simulink model "gm_HDLRx_vs"  (R2024a)
settings: Solver=FixedStepDiscrete  StartTime=0.0  StopTime=stopTime  RelTol=1e-3
undefined symbols (not defined in the file or in its folder): channelBitsPerSubcarrier, channelCyclicPrefixLen, channelOFDMSamples, channelScramblerInit, clk, clk_enable, decimatorDelay, decimatorFilter, fPHY, fs, headerBitsPerFec, headerBitsPerSubcarrier, headerCyclicPrefixLen, headerOFDMSamples, headerScramblerInit, lowerbound, N, numDataCarriers, payloadBitsPerFec, payloadScramblerInit, preambleBitsPerSubcarrier, preambleCyclicPrefixLen, preambleFirstPartOFDMSamples, preambleScramblerInit, preambleSecondPartOFDMSamples, QAM, reset_x, upperbound
libraries: hdlsllib x133, hdlmdlgenlib x132, simulink x8, whdlutilities x8, whdlmod x4, dspsrcs4 x2, whdledac x2, commhdlcrc x1, dsphdlfiltering2 x1, dsphdlsigops2 x1, vivadosimlib x1, HDL_ieee_8021513 x1
(part 1 of 4)
settings Model: Creator=cotti  LastModifiedBy=cotti
settings OptimizationCC: BlockReduction=off  ConditionallyExecuteInputs=off  DefaultParameterBehavior=Inlined  InheritOutputTypeSmallerThanSingle=on
settings DebuggingCC: AlgebraicLoopMsg=error  ArtificialAlgebraicLoopMsg=error  InheritedTsInSrcMsg=none  SingleTaskRateTransMsg=error  UnconnectedInputMsg=warning  UnconnectedOutputMsg=warning  UnconnectedLineMsg=warning
settings HardwareCC: ProdBitPerPointer=32  ProdBitPerSizeT=32  ProdBitPerPtrDiffT=32  ProdLargestAtomicFloat=None  ProdIntDivRoundTo=Undefined  ProdEndianess=Unspecified  ProdWordSize=32  ProdHWDeviceType=ASIC/FPGA->ASIC/FPGA  TargetBitPerLong=64  TargetBitPerPointer=64  TargetBitPerSizeT=64  TargetBitPerPtrDiffT=64  TargetLongLongMode=on  TargetIntDivRoundTo=Zero  TargetEndianess=LittleEndian  TargetWordSize=64  TargetHWDeviceType=Custom Processor->MATLAB Host Computer  ProdEqTarget=off

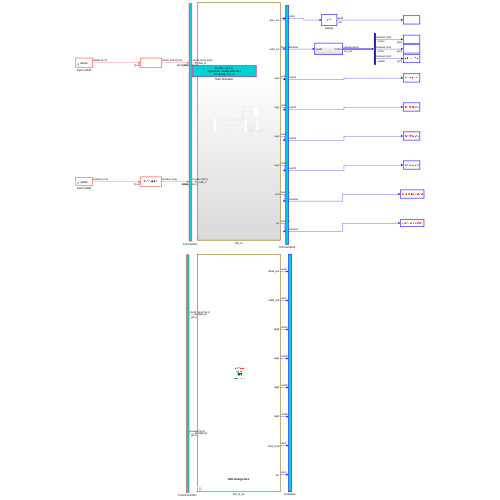
[thumbnail: Simulink's stored preview of the top-level diagram]
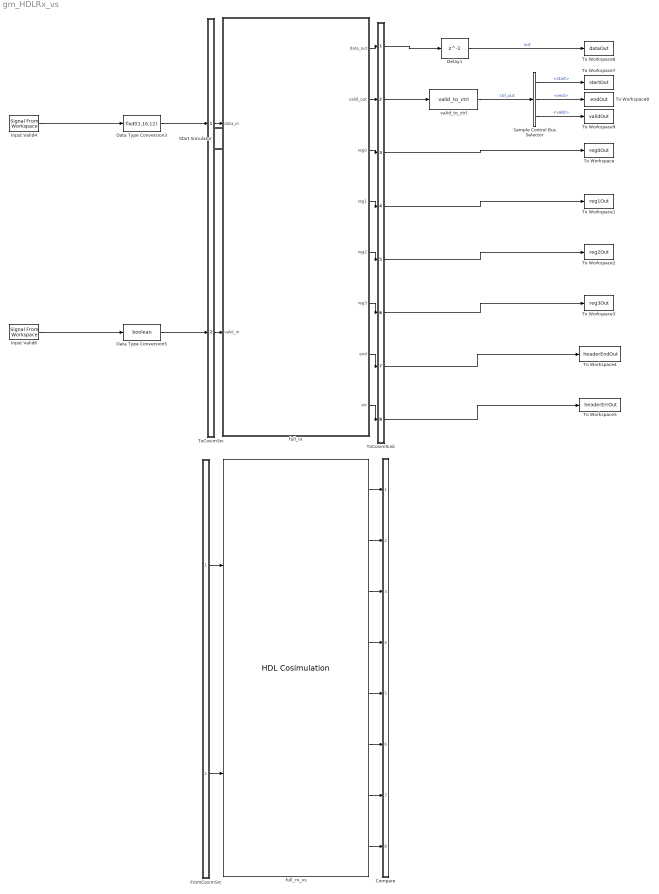
== system gm_HDLRx_vs ==
  Compare : Subsystem
      mask Display: disp('')
  Data Type Conversion3 : DataTypeConversion  OutDataTypeStr=fixdt(1,16,12)  SaturateOnIntegerOverflow=off  RndMeth=Floor
  Data Type Conversion5 : DataTypeConversion  OutDataTypeStr=boolean  SaturateOnIntegerOverflow=off  RndMeth=Floor
  Delay1 : Delay  DelayLength=1  InitialCondition=0  UseCircularBuffer=on
  FromCosimSrc : Subsystem
      mask Display: disp('')
  Input Valid4 : dspsrcs4/Signal From Workspace  X=dataIn  Ts=1/fs  nsamps=1  OutputAfterFinalValue=Setting to zero  ignoreOrWarnInputAndFrameLengths=off  OutputFrames=off
  Input Valid6 : dspsrcs4/Signal From Workspace  X=validIn  Ts=1/fs  nsamps=1  OutputAfterFinalValue=Setting to zero  ignoreOrWarnInputAndFrameLengths=off  OutputFrames=off
  Sample Control Bus Selector : whdlutilities/Sample Control Bus Selector  OutputSignals=start,end,valid
  Start Simulator : Subsystem
      settings: OpenFcn=|
      | cosimDirName = pwd;
      | cd 'hdl_prj/hdlsrc/HDLRx';
      | [s,r] = system('vivado -mode batch -source gm_HDLRx_vs.tcl','-echo');
      | cd (cosimDirName);
      | clear cosimDirName;
      | if s
      |    error('Failed to create Vivado HDL design DLL using script gm_HDLRx_vs.tcl.');
      | end
      mask Display: disp('Double-click to\nregenerate Vivado HDL DLL\nfor design full_rx')
  To Workspace : ToWorkspace  VariableName=reg0Out  SampleTime=4/fPHY
      settings: Save2DSignal=2-D array (concatenate along first dimension)
  To Workspace1 : ToWorkspace  VariableName=reg1Out  SampleTime=4/fPHY
      settings: Save2DSignal=2-D array (concatenate along first dimension)
  To Workspace2 : ToWorkspace  VariableName=reg2Out  SampleTime=4/fPHY
      settings: Save2DSignal=2-D array (concatenate along first dimension)
  To Workspace3 : ToWorkspace  VariableName=reg3Out  SampleTime=4/fPHY
      settings: Save2DSignal=2-D array (concatenate along first dimension)
  To Workspace4 : ToWorkspace  VariableName=headerEndOut  SampleTime=4/fPHY
      settings: Save2DSignal=2-D array (concatenate along first dimension)
  To Workspace5 : ToWorkspace  VariableName=headerErrOut  SampleTime=4/fPHY
      settings: Save2DSignal=2-D array (concatenate along first dimension)
  To Workspace6 : ToWorkspace  VariableName=dataOut  SampleTime=4/fPHY
      settings: Save2DSignal=2-D array (concatenate along first dimension)
  To Workspace7 : ToWorkspace  VariableName=startOut  SampleTime=4/fPHY
      settings: Save2DSignal=2-D array (concatenate along first dimension)
  To Workspace8 : ToWorkspace  VariableName=endOut  SampleTime=4/fPHY
      settings: Save2DSignal=2-D array (concatenate along first dimension)
  To Workspace9 : ToWorkspace  VariableName=validOut  SampleTime=4/fPHY
      settings: Save2DSignal=2-D array (concatenate along first dimension)
  ToCosimSink : Subsystem
      mask Display: disp('')
  ToCosimSrc : Subsystem
      mask Display: disp('')
  full_rx : Subsystem
  full_rx_vs : vivadosimlib/HDL Cosimulation  PortPaths=/full_rx/data_in;/full_rx/valid_in;/full_rx/data_out;/full_rx/valid_out;/full_rx/reg0;/full_rx/reg1;/full_rx/reg2;/full_rx/reg3;/full_rx/end_rsvd;/full_rx/err  PortModes=[1 1 2 2 2 2 2 2 2 2 ]  PortTimes=[-1 -1 8.0000000000000001673804866410277814026130727143026888370513916016e-08 8.0000000000000001673804866410277814026130727143026888370513916016e-08 8.0000000000000001673804866410277814026130727143026888370513916016e-08 8.0000000000000001673804866410277814026130727143026888370513916016e-08 8.0000000000000001673804866410277814026130727143026888370513916016e-08 8.0000000000000001673804866410277814026130727143026888370513916016e-08 8.0000000000000001673804866410277814026130727143026888370513916016e-08 8.0000000000000001673804866410277814026130727143026888370513916016e-08 ]  PortSigns=[-1 -1 0 0 0 0 0 0 0 0 ]  PortFracLengths=[0,0,0,0,0,0,0,0,0,0]  PortWordLengths=[-1,-1,8,1,32,32,32,32,1,1]  PortHDLWordSizes=[16,1,8,1,32,32,32,32,1,1]  CommLocal=on  CommSharedMemory=on  CommPortNumber=4449  CommShowInfo=on  ClockPaths=clk;clk_enable;reset_x;  ClockModes=[2 4 3]  ClockTimes=[1e-08 3.7e-08 2.7e-08]  TclPostSimCommand="puts \"done\""  TimingMode=ns  TimingScaleFactor=1000000000  idxCellArray={'UNUSED_VAR'}  CosimBypass=Full Simulation  AllowDirectFeedthrough=on  ProductName=EDA Simulator Link VS  RunAutoTimescale=off  HdlClocks=0  PreRunTime=40  PreRunTimeUnit=ns
  valid_to_ctrl : HDL_ieee_8021513/valid_to_ctrl  SystemSampleTime=-1  VariantActivationTime=update diagram  AllowFlexibleInterface=on  Latency=0  AutoFrameSizeCalculation=off
      settings: SourceProductName=HDL IEEE 8021513
  wires:
  Sample Control Bus Selector/3 -> To Workspace9/1  "<valid>"
  Sample Control Bus Selector/1 -> To Workspace7/1  "<start>"
  Delay1/1 -> To Workspace6/1  "out"
  valid_to_ctrl/1 -> Sample Control Bus Selector/1  "ctrl_out"
  Sample Control Bus Selector/2 -> To Workspace8/1  "<end>"
  Input Valid6/1 -> Data Type Conversion5/1
  Input Valid4/1 -> Data Type Conversion3/1
  ToCosimSrc/1(out1) -> full_rx/1(data_in)
  ToCosimSrc/2(out2) -> full_rx/2(valid_in)
  full_rx/1(data_out) -> ToCosimSink/1(in1)
  full_rx/2(valid_out) -> ToCosimSink/2(in2)
  full_rx/3(reg0) -> ToCosimSink/3(in3)
  full_rx/4(reg1) -> ToCosimSink/4(in4)
  full_rx/5(reg2) -> ToCosimSink/5(in5)
  full_rx/6(reg3) -> ToCosimSink/6(in6)
  full_rx/7(end) -> ToCosimSink/7(in7)
  full_rx/8(err) -> ToCosimSink/8(in8)
  Data Type Conversion3/1 -> ToCosimSrc/1(in1)
  Data Type Conversion5/1 -> ToCosimSrc/2(in2)
  ToCosimSink/1(out1) -> Delay1/1
  ToCosimSink/2(out2) -> valid_to_ctrl/1
  ToCosimSink/3(out3) -> To Workspace/1
  ToCosimSink/4(out4) -> To Workspace1/1
  ToCosimSink/5(out5) -> To Workspace2/1
  ToCosimSink/6(out6) -> To Workspace3/1
  ToCosimSink/7(out7) -> To Workspace4/1
  ToCosimSink/8(out8) -> To Workspace5/1
  FromCosimSrc/1(out1) -> full_rx_vs/1
  FromCosimSrc/2(out2) -> full_rx_vs/2
  full_rx_vs/1 -> Compare/1(in1)
  full_rx_vs/2 -> Compare/2(in2)
  full_rx_vs/3 -> Compare/3(in3)
  full_rx_vs/4 -> Compare/4(in4)
  full_rx_vs/5 -> Compare/5(in5)
  full_rx_vs/6 -> Compare/6(in6)
  full_rx_vs/7 -> Compare/7(in7)
  full_rx_vs/8 -> Compare/8(in8)

== system gm_HDLRx_vs/Compare ==
  in1 : Inport
  in2 : Inport  Port=2
  in3 : Inport  Port=3
  in4 : Inport  Port=4
  in5 : Inport  Port=5
  in6 : Inport  Port=6
  in7 : Inport  Port=7
  in8 : Inport  Port=8
  Assert_data_out : Subsystem
      settings: LibrarySourceBlock=hdlmdlgenlib/AssertEq
  Assert_end : Subsystem
      settings: LibrarySourceBlock=hdlmdlgenlib/AssertEq
  Assert_err : Subsystem
      settings: LibrarySourceBlock=hdlmdlgenlib/AssertEq
  Assert_reg0 : Subsystem
      settings: LibrarySourceBlock=hdlmdlgenlib/AssertEq
  Assert_reg1 : Subsystem
      settings: LibrarySourceBlock=hdlmdlgenlib/AssertEq
  Assert_reg2 : Subsystem
      settings: LibrarySourceBlock=hdlmdlgenlib/AssertEq
  Assert_reg3 : Subsystem
      settings: LibrarySourceBlock=hdlmdlgenlib/AssertEq
  Assert_valid_out : Subsystem
      settings: LibrarySourceBlock=hdlmdlgenlib/AssertEq
  CleanupScopes : Subsystem
      settings: OpenFcn=|
      | blkName = gcb; %self block
      | idx = regexp(blkName, '/CleanupScopes$', 'once');
      | blkParent = blkName(1:idx-1);
      | blks=find_system(blkParent, 'LookUnderMasks', 'all','blocktype', 'Scope');
      | for itr = 1:length(blks)
      | 	 hScopeCfg = get_param(blks{itr},'ScopeConfiguration');
      | 	 hScopeCfg.Visible = ~ hScopeCfg.Visible;
      | end
      | drawnow;
      mask Display: fprintf(message('hdlcoder:cosim:vnl_dblclick').getString());
  Enable : Subsystem
      settings: OpenFcn=|
      | blkName = gcb;
      | idx = regexp(blkName, '/Enable$', 'once');
      | blkParent = blkName(1:idx-1);
      | blks=find_system(blkParent, 'LookUnderMasks', 'all','blocktype', 'Assertion');
      | e = get_param(blks{1}, 'Enabled');
      | if strcmp(e, 'on'), f= 'off';, else, f = 'on';, end
      | for ii=1:length(blks), set_param(blks{ii}, 'Enabled', f);, end
      | set_param(gcb, 'MaskDisplay',['fprintf(message(''hdlcoder:cosim:vnl_dblclick_assertions'',','''',upper(e),'''',').getString())']);
      mask Display: fprintf(message('hdlcoder:cosim:vnl_dblclick_assertions','OFF').getString());
  wires:
  [out2] -> Assert_valid_out/2(dut)
  in2/1 -> Assert_valid_out/1(cosim)
  in4/1 -> Assert_reg1/1(cosim)
  [out4] -> Assert_reg1/2(dut)
  in5/1 -> Assert_reg2/1(cosim)
  [out5] -> Assert_reg2/2(dut)
  [out1] -> Assert_data_out/2(dut)
  [out7] -> Assert_end/2(dut)
  in6/1 -> Assert_reg3/1(cosim)
  [out3] -> Assert_reg0/2(dut)
  [out6] -> Assert_reg3/2(dut)
  [out8] -> Assert_err/2(dut)
  in8/1 -> Assert_err/1(cosim)
  in7/1 -> Assert_end/1(cosim)
  in1/1 -> Assert_data_out/1(cosim)
  in3/1 -> Assert_reg0/1(cosim)

== system gm_HDLRx_vs/FromCosimSrc ==
  out1 : Outport
  out2 : Outport  Port=2
  wires:
  [in2] -> out2/1
  [in1] -> out1/1

== system gm_HDLRx_vs/Start Simulator ==

== system gm_HDLRx_vs/ToCosimSink ==
  in1 : Inport
  in2 : Inport  Port=2
  in3 : Inport  Port=3
  in4 : Inport  Port=4
  in5 : Inport  Port=5
  in6 : Inport  Port=6
  in7 : Inport  Port=7
  in8 : Inport  Port=8
  out1 : Outport
  out2 : Outport  Port=2
  out3 : Outport  Port=3
  out4 : Outport  Port=4
  out5 : Outport  Port=5
  out6 : Outport  Port=6
  out7 : Outport  Port=7
  out8 : Outport  Port=8
  tag scope: out1=global, out2=global, out3=global, out4=global, out5=global, out6=global, out7=global, out8=global
  wires:
  in1/1 -> out1/1, [out1]
  in2/1 -> out2/1, [out2]
  in3/1 -> out3/1, [out3]
  in4/1 -> out4/1, [out4]
  in5/1 -> out5/1, [out5]
  in6/1 -> out6/1, [out6]
  in7/1 -> out7/1, [out7]
  in8/1 -> out8/1, [out8]

== system gm_HDLRx_vs/ToCosimSrc ==
  in1 : Inport
  in2 : Inport  Port=2
  out1 : Outport
  out2 : Outport  Port=2
  tag scope: in1=global, in2=global
  wires:
  in1/1 -> out1/1, [in1]
  in2/1 -> out2/1, [in2]

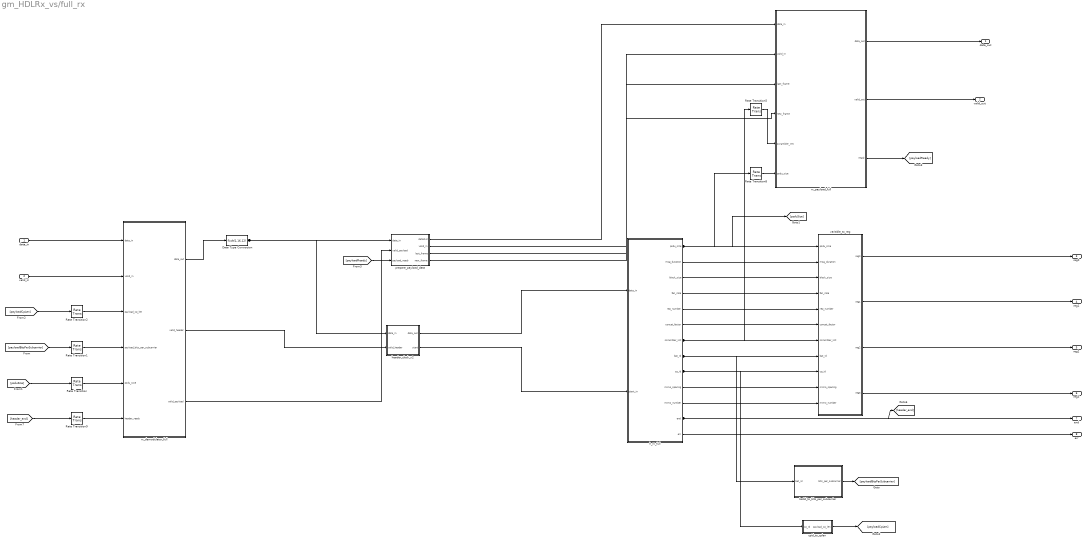
== system gm_HDLRx_vs/full_rx ==
  data_in : Inport  OutDataTypeStr=fixdt(1, 16, 12)  SampleTime=1e-08
  valid_in : Inport  Port=2  OutDataTypeStr=boolean  SampleTime=1e-08
  Data Type Conversion : DataTypeConversion  OutDataTypeStr=fixdt(1,16,12)  SaturateOnIntegerOverflow=off  RndMeth=Floor
  Rate Transition{,1..2,9} (4 alike) : RateTransition  OutPortSampleTime=1/fPHY
  Rate Transition5 : RateTransition  OutPortSampleTime=1/(2*fPHY)
  Rate Transition8 : RateTransition  OutPortSampleTime=1/(2*fPHY)
  batid_to_bits_per_subcarrier : Subsystem
  cpid_to_cplen : Subsystem
  h_rx_full : Subsystem
  header_clock_x2 : Subsystem
  prepare_payload_data : Subsystem
  rx_demodulator_full : Subsystem
  rx_payload_full : Subsystem
  variable_to_reg : Subsystem
  data_out : Outport  SampleTime=8e-08
  valid_out : Outport  Port=2  SampleTime=8e-08
  reg0 : Outport  Port=3  SampleTime=8e-08
  reg1 : Outport  Port=4  SampleTime=8e-08
  reg2 : Outport  Port=5  SampleTime=8e-08
  reg3 : Outport  Port=6  SampleTime=8e-08
  end : Outport  Port=7  SampleTime=8e-08
  err : Outport  Port=8  SampleTime=8e-08
  wires:
  variable_to_reg/4(reg3) -> reg3/1
  variable_to_reg/3(reg2) -> reg2/1
  variable_to_reg/2(reg1) -> reg1/1
  variable_to_reg/1(reg0) -> reg0/1
  rx_payload_full/3(ready) -> [payloadReady]
  rx_payload_full/2(valid_out) -> valid_out/1
  rx_payload_full/1(data_out) -> data_out/1
  rx_demodulator_full/3(valid_payload) -> prepare_payload_data/2(valid_payload)
  rx_demodulator_full/2(valid_header) -> header_clock_x2/2(valid_header)
  rx_demodulator_full/1(data_out) -> Data Type Conversion/1
  prepare_payload_data/4(new_frame) -> rx_payload_full/4(new_frame)
  prepare_payload_data/3(last_frame) -> rx_payload_full/3(last_frame)
  prepare_payload_data/2(valid_in) -> rx_payload_full/2(valid_in)
  prepare_payload_data/1(dataOut) -> rx_payload_full/1(data_in)
  header_clock_x2/2(start) -> h_rx_full/2(start_in)
  header_clock_x2/1(data_out) -> h_rx_full/1(data_in)
  h_rx_full/13(err) -> err/1
  h_rx_full/12(end) -> end/1, [header_end]
  h_rx_full/11(mimo_number) -> variable_to_reg/11(mimo_number)
  h_rx_full/10(mimo_spacing) -> variable_to_reg/10(mimo_spacing)
  h_rx_full/9(cp_id) -> cpid_to_cplen/1(cp_id), variable_to_reg/9(cp_id)
  h_rx_full/8(bat_id) -> batid_to_bits_per_subcarrier/1(bat_id), variable_to_reg/8(bat_id)
  h_rx_full/7(scrambler_init) -> variable_to_reg/7(scrambler_init), Rate Transition5/1
  h_rx_full/6(concat_factor) -> variable_to_reg/6(concat_factor)
  h_rx_full/5(rep_number) -> variable_to_reg/5(rep_number)
  h_rx_full/4(fec_rate) -> variable_to_reg/4(fec_rate)
  h_rx_full/3(block_size) -> variable_to_reg/3(block_size)
  h_rx_full/2(msg_duration) -> variable_to_reg/2(msg_duration)
  h_rx_full/1(psdu_size) -> variable_to_reg/1(psdu_size), [psduSize], Rate Transition8/1
  cpid_to_cplen/1(payload_cp_len) -> [payloadCpLen]
  batid_to_bits_per_subcarrier/1(bits_per_subcarrier) -> [payloadBitsPerSubcarrier]
  Rate Transition9/1 -> rx_demodulator_full/6(header_ready)
  Rate Transition8/1 -> rx_payload_full/6(psdu_size)
  Rate Transition5/1 -> rx_payload_full/5(scrambler_init)
  Rate Transition2/1 -> rx_demodulator_full/3(payload_cp_len)
  Rate Transition1/1 -> rx_demodulator_full/4(payload_bits_per_subcarrier)
  Rate Transition/1 -> rx_demodulator_full/5(psdu_size)
  [header_end] -> Rate Transition9/1
  [payloadReady] -> prepare_payload_data/3(payload_ready)
  [payloadCpLen] -> Rate Transition2/1
  [psduSize] -> Rate Transition/1
  [payloadBitsPerSubcarrier] -> Rate Transition1/1
  Data Type Conversion/1 -> prepare_payload_data/1(data_in), header_clock_x2/1(data_in)
  valid_in/1 -> rx_demodulator_full/2(valid_in)
  data_in/1 -> rx_demodulator_full/1(data_in)

== system gm_HDLRx_vs/Compare/Assert_data_out ==
  cosim : Inport
  dut : Inport  Port=2
  AssertEq : Assertion
  Compare To Zero : simulink/Logic and Bit Operations/Compare To Zero  relop===  OutDataTypeStr=boolean
  Relational Operator : RelationalOperator  Operator===  OutDataTypeStr=boolean  InputSameDT=off
  compare: data_out : Scope  NumInputPorts=3
  wires:
  Compare To Zero/1 -> compare: data_out/3  "err"
  Relational Operator/1 -> Compare To Zero/1, AssertEq/1
  cosim/1 -> compare: data_out/1, Relational Operator/1  "cosim"
  dut/1 -> compare: data_out/2, Relational Operator/2  "dut ref"

== system gm_HDLRx_vs/Compare/Assert_end ==
  cosim : Inport
  dut : Inport  Port=2
  AssertEq : Assertion
  Compare To Zero : simulink/Logic and Bit Operations/Compare To Zero  relop===  OutDataTypeStr=boolean
  Relational Operator : RelationalOperator  Operator===  OutDataTypeStr=boolean  InputSameDT=off
  compare: end : Scope  NumInputPorts=3
  wires:
  Compare To Zero/1 -> compare: end/3  "err"
  Relational Operator/1 -> Compare To Zero/1, AssertEq/1
  cosim/1 -> compare: end/1, Relational Operator/1  "cosim"
  dut/1 -> compare: end/2, Relational Operator/2  "dut ref"

== system gm_HDLRx_vs/Compare/Assert_err ==
  cosim : Inport
  dut : Inport  Port=2
  AssertEq : Assertion
  Compare To Zero : simulink/Logic and Bit Operations/Compare To Zero  relop===  OutDataTypeStr=boolean
  Relational Operator : RelationalOperator  Operator===  OutDataTypeStr=boolean  InputSameDT=off
  compare: err : Scope  NumInputPorts=3
  wires:
  Compare To Zero/1 -> compare: err/3  "err"
  Relational Operator/1 -> Compare To Zero/1, AssertEq/1
  cosim/1 -> compare: err/1, Relational Operator/1  "cosim"
  dut/1 -> compare: err/2, Relational Operator/2  "dut ref"

== system gm_HDLRx_vs/Compare/Assert_reg0 ==
  cosim : Inport
  dut : Inport  Port=2
  AssertEq : Assertion
  Compare To Zero : simulink/Logic and Bit Operations/Compare To Zero  relop===  OutDataTypeStr=boolean
  Relational Operator : RelationalOperator  Operator===  OutDataTypeStr=boolean  InputSameDT=off
  compare: reg0 : Scope  NumInputPorts=3
  wires:
  Compare To Zero/1 -> compare: reg0/3  "err"
  Relational Operator/1 -> Compare To Zero/1, AssertEq/1
  cosim/1 -> compare: reg0/1, Relational Operator/1  "cosim"
  dut/1 -> compare: reg0/2, Relational Operator/2  "dut ref"

== system gm_HDLRx_vs/Compare/Assert_reg1 ==
  cosim : Inport
  dut : Inport  Port=2
  AssertEq : Assertion
  Compare To Zero : simulink/Logic and Bit Operations/Compare To Zero  relop===  OutDataTypeStr=boolean
  Relational Operator : RelationalOperator  Operator===  OutDataTypeStr=boolean  InputSameDT=off
  compare: reg1 : Scope  NumInputPorts=3
  wires:
  Compare To Zero/1 -> compare: reg1/3  "err"
  Relational Operator/1 -> Compare To Zero/1, AssertEq/1
  cosim/1 -> compare: reg1/1, Relational Operator/1  "cosim"
  dut/1 -> compare: reg1/2, Relational Operator/2  "dut ref"

== system gm_HDLRx_vs/Compare/Assert_reg2 ==
  cosim : Inport
  dut : Inport  Port=2
  AssertEq : Assertion
  Compare To Zero : simulink/Logic and Bit Operations/Compare To Zero  relop===  OutDataTypeStr=boolean
  Relational Operator : RelationalOperator  Operator===  OutDataTypeStr=boolean  InputSameDT=off
  compare: reg2 : Scope  NumInputPorts=3
  wires:
  Compare To Zero/1 -> compare: reg2/3  "err"
  Relational Operator/1 -> Compare To Zero/1, AssertEq/1
  cosim/1 -> compare: reg2/1, Relational Operator/1  "cosim"
  dut/1 -> compare: reg2/2, Relational Operator/2  "dut ref"

== system gm_HDLRx_vs/Compare/Assert_reg3 ==
  cosim : Inport
  dut : Inport  Port=2
  AssertEq : Assertion
  Compare To Zero : simulink/Logic and Bit Operations/Compare To Zero  relop===  OutDataTypeStr=boolean
  Relational Operator : RelationalOperator  Operator===  OutDataTypeStr=boolean  InputSameDT=off
  compare: reg3 : Scope  NumInputPorts=3
  wires:
  Compare To Zero/1 -> compare: reg3/3  "err"
  Relational Operator/1 -> Compare To Zero/1, AssertEq/1
  cosim/1 -> compare: reg3/1, Relational Operator/1  "cosim"
  dut/1 -> compare: reg3/2, Relational Operator/2  "dut ref"

== system gm_HDLRx_vs/Compare/Assert_valid_out ==
  cosim : Inport
  dut : Inport  Port=2
  AssertEq : Assertion
  Compare To Zero : simulink/Logic and Bit Operations/Compare To Zero  relop===  OutDataTypeStr=boolean
  Relational Operator : RelationalOperator  Operator===  OutDataTypeStr=boolean  InputSameDT=off
  compare: valid_out : Scope  NumInputPorts=3
  wires:
  Compare To Zero/1 -> compare: valid_out/3  "err"
  Relational Operator/1 -> Compare To Zero/1, AssertEq/1
  cosim/1 -> compare: valid_out/1, Relational Operator/1  "cosim"
  dut/1 -> compare: valid_out/2, Relational Operator/2  "dut ref"

== system gm_HDLRx_vs/Compare/CleanupScopes ==

== system gm_HDLRx_vs/Compare/Enable ==

== system gm_HDLRx_vs/full_rx/batid_to_bits_per_subcarrier ==
  note: Remember that "bat_id" is LSB first.
  note: De momento, el valor de BATID va a coincidir con el valor de la cantidad de bits por subcarrier.
  bat_id : Inport  OutDataTypeStr=fixdt(0, 1, 0)  PortDimensions=[5]  SampleTime=8e-08
  Bit Concat : hdlsllib/Logic and Bit Operations/Bit Concat  numInputs=4
  From{,1..3} (4 alike) : hdlmdlgenlib/Buffer
  Goto{1..4} (4 alike) : hdlmdlgenlib/Buffer
  bat_id_4_term4 : Terminator
  t : Demux  Outputs=5
  bits_per_subcarrier : Outport  SampleTime=8e-08
  wires:
  t/5 -> bat_id_4_term4/1
  t/4 -> Goto1/1
  t/3 -> Goto2/1
  t/2 -> Goto3/1
  t/1 -> Goto4/1
  Goto1/1 -> From3/1
  Goto2/1 -> From2/1
  Goto3/1 -> From1/1
  Goto4/1 -> From/1
  From3/1 -> Bit Concat/1
  From2/1 -> Bit Concat/2
  From1/1 -> Bit Concat/3
  From/1 -> Bit Concat/4
  Bit Concat/1 -> bits_per_subcarrier/1
  bat_id/1 -> t/1

== system gm_HDLRx_vs/full_rx/cpid_to_cplen ==
  cp_id : Inport  OutDataTypeStr=fixdt(0, 1, 0)  PortDimensions=[3]  SampleTime=8e-08
  Bits to Word : hdlsllib/Logic and Bit Operations/Bits to Word
  Constant3 : Constant  Value=N/32  OutDataTypeStr=fixdt(0,4,0)  SampleTime=-1
  Data Type Conversion : DataTypeConversion  OutDataTypeStr=fixdt(0,1,0)  SaturateOnIntegerOverflow=off  RndMeth=Floor
  Delay1 : Delay  DelayLength=1  InitialCondition=0  UseCircularBuffer=on
  Product : Product  OutDataTypeStr=uint8
  payload_cp_len : Outport  SampleTime=8e-08
  wires:
  Product/1 -> Delay1/1
  Delay1/1 -> payload_cp_len/1
  Data Type Conversion/1 -> Bits to Word/1
  Constant3/1 -> Product/1
  Bits to Word/1 -> Product/2
  cp_id/1 -> Data Type Conversion/1

== system gm_HDLRx_vs/full_rx/h_rx_full ==
  data_in : Inport  OutDataTypeStr=fixdt(1, 16, 12)  SampleTime=1e-08
  start_in : Inport  Port=2  OutDataTypeStr=boolean  SampleTime=1e-08
  Data Type Conversion : DataTypeConversion  OutDataTypeStr=int8  SaturateOnIntegerOverflow=off  RndMeth=Floor
  Data Type Conversion1 : DataTypeConversion  OutDataTypeStr=boolean  SaturateOnIntegerOverflow=off  RndMeth=Floor
  LDPC_Deco_Hc_12H : whdledac/LDPC Decoder  ParityCheckMatrix=Hc_12H  BlockSize=14  Algorithm=Min-sum  ScalingFactor=0.75  Termination=Max  SpecifyInputs=Property  NumIterations=ldpcDecoderMaxNumberIterations  MaxNumIterations=8  ParityCheckStatus=off  SimulateUsing=Code generation
  LDPC_Deco_Hc_12H_term2 : Terminator
  Rate Transition : RateTransition  OutPortSampleTimeOpt=Multiple of input port sample time  OutPortSampleTimeMultiple=8
  h_crc_rx : Subsystem
  h_remove_repetition : Subsystem
  h_scrambler : Subsystem
  h_separate : Subsystem
  psdu_size : Outport  SampleTime=8e-08
  msg_duration : Outport  Port=2  SampleTime=8e-08
  block_size : Outport  Port=3  SampleTime=8e-08
  fec_rate : Outport  Port=4  SampleTime=8e-08
  rep_number : Outport  Port=5  SampleTime=8e-08
  concat_factor : Outport  Port=6  SampleTime=8e-08
  scrambler_init : Outport  Port=7  SampleTime=8e-08
  bat_id : Outport  Port=8  SampleTime=8e-08
  cp_id : Outport  Port=9  SampleTime=8e-08
  mimo_spacing : Outport  Port=10  SampleTime=8e-08
  mimo_number : Outport  Port=11  SampleTime=8e-08
  end : Outport  Port=12  SampleTime=8e-08
  err : Outport  Port=13  SampleTime=8e-08
  wires:
  h_separate/12(end) -> end/1
  h_separate/11(mimo_number) -> mimo_number/1
  h_separate/10(mimo_spacing) -> mimo_spacing/1
  h_separate/9(cp_id) -> cp_id/1
  h_separate/8(bat_id) -> bat_id/1
  h_separate/7(scrambler_init) -> scrambler_init/1
  h_separate/6(concat_factor) -> concat_factor/1
  h_separate/5(rep_number) -> rep_number/1
  h_separate/4(fec_rate) -> fec_rate/1
  h_separate/3(block_size) -> block_size/1
  h_separate/2(msg_duration) -> msg_duration/1
  h_separate/1(psdu_size) -> psdu_size/1
  h_scrambler/2(ctrl_out) -> h_crc_rx/2(ctrl_in)
  h_scrambler/1(data_out) -> h_crc_rx/1(data_in)
  h_remove_repetition/2(ctrl_out) -> LDPC_Deco_Hc_12H/2
  h_remove_repetition/1(data_out) -> LDPC_Deco_Hc_12H/1
  h_crc_rx/3(err) -> Rate Transition/1
  h_crc_rx/2(ctrl_out) -> h_separate/2(ctrl_in)
  h_crc_rx/1(data_out) -> h_separate/1(data_in)
  Rate Transition/1 -> err/1
  LDPC_Deco_Hc_12H/3 -> LDPC_Deco_Hc_12H_term2/1
  LDPC_Deco_Hc_12H/2 -> h_scrambler/2(ctrl_in)
  LDPC_Deco_Hc_12H/1 -> h_scrambler/1(data_in)
  Data Type Conversion1/1 -> h_remove_repetition/2(start_in)
  Data Type Conversion/1 -> h_remove_repetition/1(data_in)
  start_in/1 -> Data Type Conversion1/1
  data_in/1 -> Data Type Conversion/1

== system gm_HDLRx_vs/full_rx/header_clock_x2 ==
  data_in : Inport  OutDataTypeStr=fixdt(1, 16, 12)  PortDimensions=[4 1]  SampleTime=2e-08
  valid_header : Inport  Port=2  OutDataTypeStr=boolean  PortDimensions=1  SampleTime=2e-08
  Serializer1D : hdlsllib/HDL Operations/Serializer1D  Ratio=2  IdleCycles=0  validIn=on  startOut=off  validOut=on  inputDataDimensions=2  inputSampleTime=2e-08  inputSignalType=real
  concatenate : Concatenate  Mode=Multidimensional array  ConcatenateDimension=2
  data_in_0_term0 : Terminator
  data_in_1_term1 : Terminator
  rising_edge_detector : Subsystem
  t : Demux
  data_out : Outport  SampleTime=1e-08
  start : Outport  Port=2  SampleTime=1e-08
  wires:
  t/4 -> concatenate/2
  t/3 -> concatenate/1
  t/2 -> data_in_1_term1/1
  t/1 -> data_in_0_term0/1
  rising_edge_detector/1(Out) -> start/1
  concatenate/1 -> Serializer1D/1
  Serializer1D/2 -> rising_edge_detector/1(In)
  Serializer1D/1 -> data_out/1
  valid_header/1 -> Serializer1D/2
  data_in/1 -> t/1

== system gm_HDLRx_vs/full_rx/prepare_payload_data ==
  note: Note_ this delay makes sure that the fifo always has data, and is not emptied in the middle of an LDPC block
  data_in : Inport  OutDataTypeStr=fixdt(1, 16, 12)  PortDimensions=[4 1]  SampleTime=2e-08
  valid_payload : Inport  Port=2  OutDataTypeStr=boolean  PortDimensions=1  SampleTime=2e-08
  payload_ready : Inport  Port=3  OutDataTypeStr=boolean  PortDimensions=1  SampleTime=1e-08
  Delay : Delay  DelayLength=1  InitialCondition=0  UseCircularBuffer=on
  Delay2 : Delay  DelayLength=1000  InitialCondition=0  UseCircularBuffer=on
  HDL FIFO : hdlsllib/HDL RAMs/HDL FIFO  fifo_size=65536  mode=Classic  ratio=1  push_msg=Error  pop_msg=Error  show_empty=on  show_full=off  show_num=off  LabelModeActiveChoice_Mode=Classic  rst_port=off
  Logical Operator2 : Logic  IconShape=distinctive  AllPortsSameDT=off  OutDataTypeStr=boolean
  Logical Operator3 : Logic  Operator=NOT  IconShape=distinctive  AllPortsSameDT=off  OutDataTypeStr=boolean
  Rate Transition3 : RateTransition  OutPortSampleTime=1/(2*fPHY)
  Rate Transition4 : RateTransition  OutPortSampleTime=1/(2*fPHY)
  falling_edge_detector : Subsystem
  payload_clock_x2 : Subsystem
  rising_edge_detector : Subsystem
  dataOut : Outport  SampleTime=1e-08
  valid_in : Outport  Port=2  SampleTime=1e-08
  last_frame : Outport  Port=3  SampleTime=1e-08
  new_frame : Outport  Port=4  SampleTime=1e-08
  wires:
  rising_edge_detector/1(Out) -> Rate Transition3/1
  payload_clock_x2/2(valid_out) -> HDL FIFO/2
  payload_clock_x2/1(data_out) -> HDL FIFO/1
  falling_edge_detector/1(out) -> Delay2/1
  Rate Transition4/1 -> new_frame/1
  Rate Transition3/1 -> last_frame/1
  Logical Operator3/1 -> Logical Operator2/1
  Logical Operator2/1 -> HDL FIFO/3, Delay/1
  HDL FIFO/2 -> rising_edge_detector/1(In), falling_edge_detector/1(in), Logical Operator3/1
  HDL FIFO/1 -> dataOut/1
  Delay2/1 -> Rate Transition4/1
  Delay/1 -> valid_in/1
  payload_ready/1 -> Logical Operator2/2
  valid_payload/1 -> payload_clock_x2/2(valid_in)
  data_in/1 -> payload_clock_x2/1(data_in)

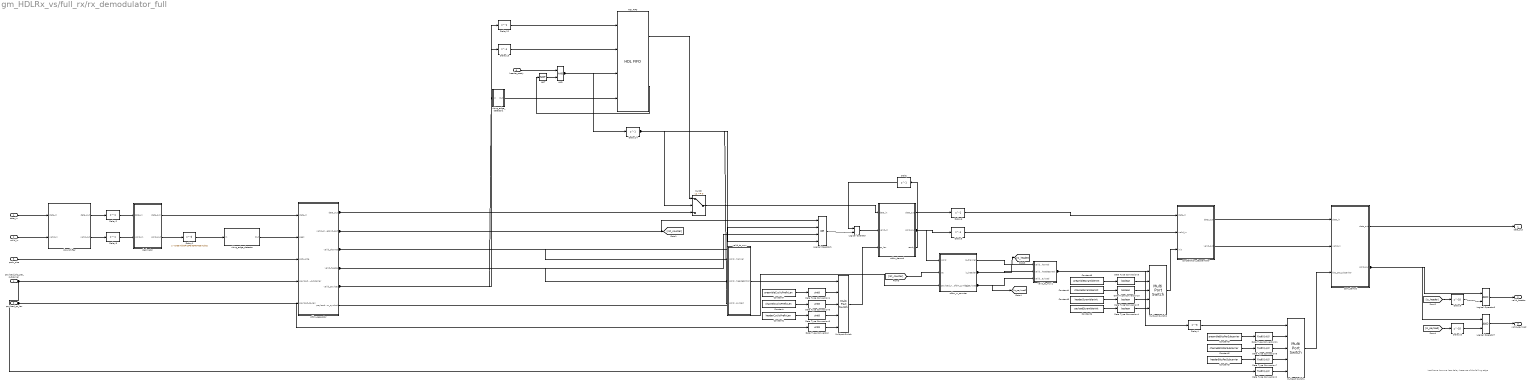
== system gm_HDLRx_vs/full_rx/rx_demodulator_full ==
  note: Last frame has one less delay because of the falling edge
  data_in : Inport  OutDataTypeStr=fixdt(1, 16, 12)  SampleTime=1e-08
  valid_in : Inport  Port=2  OutDataTypeStr=boolean  SampleTime=1e-08
  payload_cp_len : Inport  Port=3  OutDataTypeStr=uint8  SampleTime=2e-08
  payload_bits_per_subcarrier : Inport  Port=4  OutDataTypeStr=fixdt(0, 4, 0)  SampleTime=2e-08
  psdu_size : Inport  Port=5  OutDataTypeStr=fixdt(0, 1, 0)  PortDimensions=[24]  SampleTime=2e-08
  header_ready : Inport  Port=6  OutDataTypeStr=boolean  SampleTime=2e-08
  AND : Logic  IconShape=distinctive  AllPortsSameDT=off  OutDataTypeStr=boolean
  Constant : Constant  Value=channelCyclicPrefixLen  OutDataTypeStr=uint8  SampleTime=-1
  Constant1 : Constant  Value=headerCyclicPrefixLen  OutDataTypeStr=uint8  SampleTime=-1
  Constant2 : Constant  Value=channelBitsPerSubcarrier  OutDataTypeStr=uint8  SampleTime=-1
  Constant3 : Constant  Value=headerBitsPerSubcarrier  OutDataTypeStr=uint8  SampleTime=-1
  Constant4 : Constant  Value=channelScramblerInit  OutDataTypeStr=uint8  SampleTime=-1
  Constant5 : Constant  Value=headerScramblerInit  OutDataTypeStr=uint8  SampleTime=-1
  Constant6 : Constant  Value=payloadScramblerInit  OutDataTypeStr=uint8  SampleTime=-1
  Constant7 : Constant  Value=preambleCyclicPrefixLen  OutDataTypeStr=uint8  SampleTime=-1
  Constant8 : Constant  Value=preambleScramblerInit  OutDataTypeStr=uint8  SampleTime=-1
  Constant9 : Constant  Value=preambleBitsPerSubcarrier  OutDataTypeStr=uint8  SampleTime=-1
  Data Type Conversion{,1,5..6} (4 alike) : DataTypeConversion  OutDataTypeStr=uint8  SaturateOnIntegerOverflow=off  RndMeth=Floor
  Data Type Conversion{3..4,9..10} (4 alike) : DataTypeConversion  OutDataTypeStr=boolean  SaturateOnIntegerOverflow=off  RndMeth=Floor
  Data Type Conversion{2,7..8,11} (4 alike) : DataTypeConversion  OutDataTypeStr=fixdt(0,4,0)  SaturateOnIntegerOverflow=off  RndMeth=Floor
  Delay{,2..3,5..6,12..14} (8 alike) : Delay  DelayLength=1  InitialCondition=0  UseCircularBuffer=on
  Delay1 : Delay  DelayLength=preambleFirstPartOFDMSamples  InitialCondition=0  UseCircularBuffer=on
  Delay10 : Delay  DelayLength=10  InitialCondition=0  UseCircularBuffer=on
  Delay4 : Delay  DelayLength=3  InitialCondition=0  UseCircularBuffer=on
  Delay9 : Delay  DelayLength=10  InitialCondition=0  UseCircularBuffer=on
  HDL FIFO : hdlsllib/HDL RAMs/HDL FIFO  fifo_size=8192  mode=Classic  ratio=1  push_msg=Error  pop_msg=Error  show_empty=on  show_full=off  show_num=off  LabelModeActiveChoice_Mode=Classic  rst_port=on
  Logical Operator : Logic  IconShape=distinctive  AllPortsSameDT=off  OutDataTypeStr=boolean
  Logical Operator1 : Logic  Operator=OR  Inputs=4  IconShape=distinctive  AllPortsSameDT=off  OutDataTypeStr=boolean
  Logical Operator6 : Logic  IconShape=distinctive  AllPortsSameDT=off  OutDataTypeStr=boolean
  Logical Operator7 : Logic  IconShape=distinctive  AllPortsSameDT=off  OutDataTypeStr=boolean
  Multiport Switch : MultiPortSwitch  DataPortOrder=Zero-based contiguous  Inputs=4  zeroidx=on  OutDataTypeStr=uint8  SaturateOnIntegerOverflow=off  InputSameDT=off
  Multiport Switch1 : MultiPortSwitch  DataPortOrder=Zero-based contiguous  Inputs=4  zeroidx=on  OutDataTypeStr=fixdt(0, 4, 0)  SaturateOnIntegerOverflow=off  InputSameDT=off
  Multiport Switch2 : MultiPortSwitch  DataPortOrder=Zero-based contiguous  Inputs=4  zeroidx=on  SaturateOnIntegerOverflow=off  InputSameDT=off
  NOT : Logic  Operator=NOT  IconShape=distinctive  AllPortsSameDT=off  OutDataTypeStr=boolean
  Switch : Switch  Criteria=u2 ~= 0  OutDataTypeStr=fixdt(1, 16, 12)  SaturateOnIntegerOverflow=off  InputSameDT=off
  constellation_descrambler : Subsystem
  decimator : Subsystem
  downshifter : Subsystem
  ofdm_demod : Subsystem
  ofdm_rx_counter : Subsystem
  ofdm_separator : Subsystem
  qam_demod : Subsystem
  rising_edge_detector : Subsystem
  rising_edge_detector1 : Subsystem
  valid_to_mux : Subsystem
  valid_to_mux1 : Subsystem
  data_out : Outport  SampleTime=2e-08
  valid_header : Outport  Port=2  SampleTime=2e-08
  valid_payload : Outport  Port=3  SampleTime=2e-08
  wires:
  valid_to_mux1/1(control) -> Delay4/1, Multiport Switch2/1
  valid_to_mux/1(control) -> Multiport Switch/1
  rising_edge_detector1/1(Out) -> HDL FIFO/4
  rising_edge_detector/1(Out) -> ofdm_separator/2(peak)
  qam_demod/2(valid_out) -> Logical Operator6/1, Logical Operator7/1
  qam_demod/1(data_out) -> data_out/1
  ofdm_separator/6(payload_num_ofdm_symbols) -> ofdm_rx_counter/3(payload_num_ofdm_symbols)
  ofdm_separator/5(valid_payload) -> rising_edge_detector1/1(In), Delay13/1
  ofdm_separator/4(valid_header) -> valid_to_mux/2(valid_header), Logical Operator1/3
  ofdm_separator/3(valid_channel) -> valid_to_mux/1(valid_channel), Logical Operator1/2
  ofdm_separator/2(valid_preamble_second_part) -> [rst_counter], Logical Operator1/1
  ofdm_separator/1(data_out) -> Delay12/1, Switch/3
  ofdm_rx_counter/3(is_payload) -> valid_to_mux1/3(valid_payload), [is_payload]
  ofdm_rx_counter/2(is_header) -> valid_to_mux1/2(valid_header), [is_header]
  ofdm_rx_counter/1(is_channel) -> valid_to_mux1/1(valid_channel)
  ofdm_demod/3(ready) -> Delay/1
  ofdm_demod/2(valid_out) -> ofdm_rx_counter/1(valid), Delay5/1
  ofdm_demod/1(data_out) -> Delay6/1
  downshifter/2(valid_out) -> Delay3/1
  downshifter/1(data_out) -> Delay2/1
  decimator/2(valid_out) -> Delay1/1
  decimator/1(data_out) -> ofdm_separator/1(data_in)
  constellation_descrambler/2(valid_out) -> qam_demod/2(valid_in)
  constellation_descrambler/1(data_out) -> qam_demod/1(data_in)
  Switch/1 -> ofdm_demod/1(data_in)
  NOT/1 -> AND/2
  Multiport Switch2/1 -> constellation_descrambler/3(init)
  Multiport Switch1/1 -> qam_demod/3(bits_per_subcarrier)
  Multiport Switch/1 -> ofdm_demod/3(cp_len)
  Logical Operator7/1 -> valid_payload/1
  Logical Operator6/1 -> valid_header/1
  Logical Operator1/1 -> Logical Operator/2
  Logical Operator/1 -> ofdm_demod/2(valid_in)
  HDL FIFO/2 -> NOT/1
  HDL FIFO/1 -> Switch/1
  [is_payload] -> Delay10/1
  [rst_counter] -> ofdm_rx_counter/2(rst)
  [is_header] -> Delay9/1
  Delay9/1 -> Logical Operator6/2
  Delay6/1 -> constellation_descrambler/1(data_in)
  Delay5/1 -> constellation_descrambler/2(valid_in)
  Delay4/1 -> Multiport Switch1/1
  Delay3/1 -> decimator/2(valid_in)
  Delay2/1 -> decimator/1(data_in)
  Delay14/1 -> valid_to_mux/3(valid_payload), Logical Operator1/4, Switch/2
  Delay13/1 -> HDL FIFO/2
  Delay12/1 -> HDL FIFO/1
  Delay10/1 -> Logical Operator7/2
  Delay1/1 -> rising_edge_detector/1(In)
  Delay/1 -> Logical Operator/1
  Data Type Conversion9/1 -> Multiport Switch2/4
  Data Type Conversion8/1 -> Multiport Switch1/3
  Data Type Conversion7/1 -> Multiport Switch1/4
  Data Type Conversion6/1 -> Multiport Switch/3
  Data Type Conversion5/1 -> Multiport Switch/4
  Data Type Conversion4/1 -> Multiport Switch2/5
  Data Type Conversion3/1 -> Multiport Switch2/2
  Data Type Conversion2/1 -> Multiport Switch1/5
  Data Type Conversion11/1 -> Multiport Switch1/2
  Data Type Conversion10/1 -> Multiport Switch2/3
  Data Type Conversion1/1 -> Multiport Switch/2
  Data Type Conversion/1 -> Multiport Switch/5
  Constant9/1 -> Data Type Conversion11/1
  Constant8/1 -> Data Type Conversion3/1
  Constant7/1 -> Data Type Conversion1/1
  Constant6/1 -> Data Type Conversion4/1
  Constant5/1 -> Data Type Conversion9/1
  Constant4/1 -> Data Type Conversion10/1
  Constant3/1 -> Data Type Conversion7/1
  Constant2/1 -> Data Type Conversion8/1
  Constant1/1 -> Data Type Conversion5/1
  Constant/1 -> Data Type Conversion6/1
  AND/1 -> HDL FIFO/3, Delay14/1
  header_ready/1 -> AND/1
  psdu_size/1 -> ofdm_separator/3(psdu_size)
  payload_bits_per_subcarrier/1 -> ofdm_separator/4(payload_bits_per_subcarrier), Data Type Conversion2/1
  payload_cp_len/1 -> ofdm_separator/5(payload_cp_len), Data Type Conversion/1
  valid_in/1 -> downshifter/2(valid_in)
  data_in/1 -> downshifter/1(data_in)

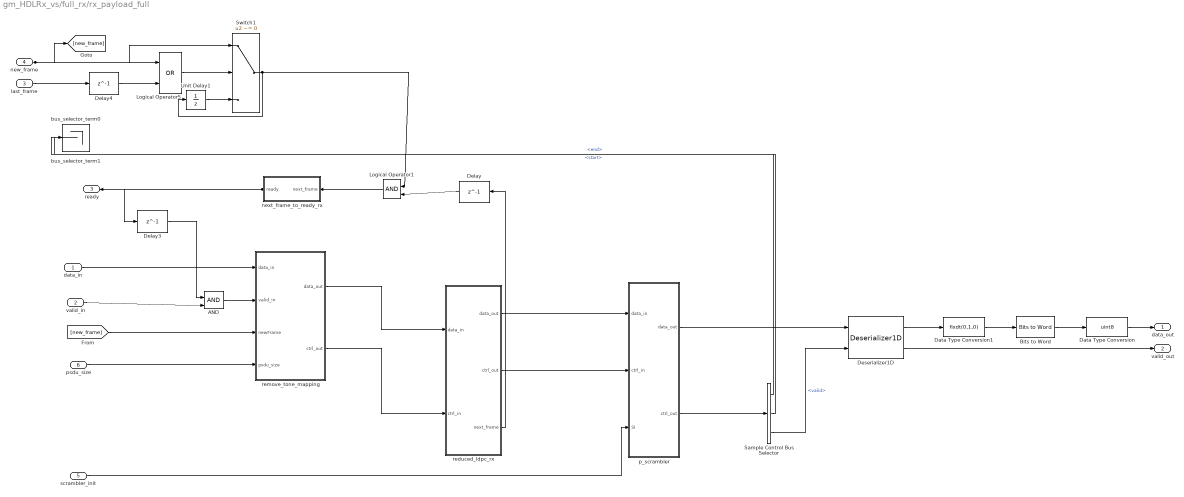
== system gm_HDLRx_vs/full_rx/rx_payload_full ==
  data_in : Inport  OutDataTypeStr=fixdt(1, 16, 12)  SampleTime=1e-08
  valid_in : Inport  Port=2  OutDataTypeStr=boolean  SampleTime=1e-08
  last_frame : Inport  Port=3  OutDataTypeStr=boolean  SampleTime=1e-08
  new_frame : Inport  Port=4  OutDataTypeStr=boolean  SampleTime=1e-08
  scrambler_init : Inport  Port=5  OutDataTypeStr=fixdt(0, 1, 0)  PortDimensions=[4]  SampleTime=1e-08
  psdu_size : Inport  Port=6  OutDataTypeStr=fixdt(0, 1, 0)  PortDimensions=[24]  SampleTime=1e-08
  AND : Logic  IconShape=distinctive  AllPortsSameDT=off  OutDataTypeStr=boolean
  Bits to Word : hdlsllib/Logic and Bit Operations/Bits to Word
  Data Type Conversion : DataTypeConversion  OutDataTypeStr=uint8  SaturateOnIntegerOverflow=off  RndMeth=Floor
  Data Type Conversion1 : DataTypeConversion  OutDataTypeStr=fixdt(0,1,0)  SaturateOnIntegerOverflow=off  RndMeth=Floor
  Delay : Delay  DelayLength=1  InitialCondition=0  UseCircularBuffer=on
  Delay3 : Delay  DelayLength=1  InitialCondition=0  UseCircularBuffer=on
  Delay4 : Delay  DelayLength=1  InitialCondition=0  UseCircularBuffer=on
  Deserializer1D : hdlsllib/HDL Operations/Deserializer1D  Ratio=8  IdleCycles=0  InitialCondition=0  startIn=off  validIn=on  validOut=on  inputDataDimensions=-1  inputSampleTime=-1  inputSignalType=auto
  Logical Operator1 : Logic  IconShape=distinctive  AllPortsSameDT=off  OutDataTypeStr=boolean
  Logical Operator5 : Logic  Operator=OR  IconShape=distinctive  AllPortsSameDT=off  OutDataTypeStr=boolean
  Sample Control Bus Selector : whdlutilities/Sample Control Bus Selector  OutputSignals=start,end,valid
  Switch1 : Switch  Criteria=u2 ~= 0  OutDataTypeStr=boolean  SaturateOnIntegerOverflow=off  InputSameDT=off
  Unit Delay1 : UnitDelay  SampleTime=-1  HasFrameUpgradeWarning=on
  bus_selector_term0 : Terminator
  bus_selector_term1 : Terminator
  next_frame_to_ready_rx : Subsystem
  p_scrambler : Subsystem
  reduced_ldpc_rx : Subsystem
  remove_tone_mapping : Subsystem
  data_out : Outport  SampleTime=8e-08
  valid_out : Outport  Port=2  SampleTime=8e-08
  ready : Outport  Port=3  SampleTime=1e-08
  wires:
  remove_tone_mapping/2(ctrl_out) -> reduced_ldpc_rx/2(ctrl_in)
  remove_tone_mapping/1(data_out) -> reduced_ldpc_rx/1(data_in)
  reduced_ldpc_rx/3(next_frame) -> Delay/1
  reduced_ldpc_rx/2(ctrl_out) -> p_scrambler/2(ctrl_in)
  reduced_ldpc_rx/1(data_out) -> p_scrambler/1(data_in)
  p_scrambler/2(ctrl_out) -> Sample Control Bus Selector/1
  p_scrambler/1(data_out) -> Deserializer1D/1
  next_frame_to_ready_rx/1(ready) -> ready/1, Delay3/1
  Unit Delay1/1 -> Switch1/3
  Switch1/1 -> Unit Delay1/1, Logical Operator1/1
  Sample Control Bus Selector/3 -> Deserializer1D/2  "<valid>"
  Sample Control Bus Selector/2 -> bus_selector_term1/1  "<end>"
  Sample Control Bus Selector/1 -> bus_selector_term0/1  "<start>"
  Logical Operator5/1 -> Switch1/2
  Logical Operator1/1 -> next_frame_to_ready_rx/1(next_frame)
  [new_frame] -> remove_tone_mapping/3(newFrame)
  Deserializer1D/2 -> valid_out/1
  Deserializer1D/1 -> Data Type Conversion1/1
  Delay4/1 -> Logical Operator5/2
  Delay3/1 -> AND/1
  Delay/1 -> Logical Operator1/2
  Data Type Conversion1/1 -> Bits to Word/1
  Data Type Conversion/1 -> data_out/1
  Bits to Word/1 -> Data Type Conversion/1
  AND/1 -> remove_tone_mapping/2(valid_in)
  psdu_size/1 -> remove_tone_mapping/4(psdu_size)
  scrambler_init/1 -> p_scrambler/3(SI)
  new_frame/1 -> [new_frame], Logical Operator5/1, Switch1/1
  last_frame/1 -> Delay4/1
  valid_in/1 -> AND/2
  data_in/1 -> remove_tone_mapping/1(data_in)

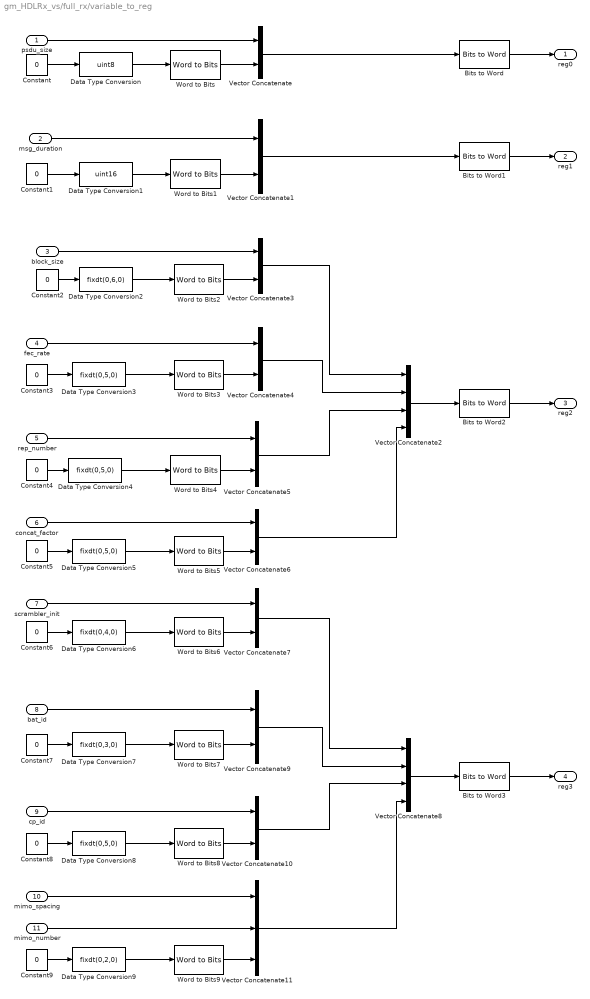
== system gm_HDLRx_vs/full_rx/variable_to_reg ==
  psdu_size : Inport  OutDataTypeStr=fixdt(0, 1, 0)  PortDimensions=[24]  SampleTime=8e-08
  msg_duration : Inport  Port=2  OutDataTypeStr=fixdt(0, 1, 0)  PortDimensions=[16]  SampleTime=8e-08
  block_size : Inport  Port=3  OutDataTypeStr=fixdt(0, 1, 0)  PortDimensions=[2]  SampleTime=8e-08
  fec_rate : Inport  Port=4  OutDataTypeStr=fixdt(0, 1, 0)  PortDimensions=[3]  SampleTime=8e-08
  rep_number : Inport  Port=5  OutDataTypeStr=fixdt(0, 1, 0)  PortDimensions=[3]  SampleTime=8e-08
  concat_factor : Inport  Port=6  OutDataTypeStr=fixdt(0, 1, 0)  PortDimensions=[3]  SampleTime=8e-08
  scrambler_init : Inport  Port=7  OutDataTypeStr=fixdt(0, 1, 0)  PortDimensions=[4]  SampleTime=8e-08
  bat_id : Inport  Port=8  OutDataTypeStr=fixdt(0, 1, 0)  PortDimensions=[5]  SampleTime=8e-08
  cp_id : Inport  Port=9  OutDataTypeStr=fixdt(0, 1, 0)  PortDimensions=[3]  SampleTime=8e-08
  mimo_spacing : Inport  Port=10  OutDataTypeStr=fixdt(0, 1, 0)  PortDimensions=[3]  SampleTime=8e-08
  mimo_number : Inport  Port=11  OutDataTypeStr=fixdt(0, 1, 0)  PortDimensions=[3]  SampleTime=8e-08
  Bits to Word{,1..3} (4 alike) : hdlsllib/Logic and Bit Operations/Bits to Word
  Constant : Constant  Value=0  OutDataTypeStr=uint8  SampleTime=-1
  Constant1 : Constant  Value=0  OutDataTypeStr=uint16  SampleTime=-1
  Constant2 : Constant  Value=0  OutDataTypeStr=fixdt(0,6,0)  SampleTime=-1
  Constant{3..5,8} (4 alike) : Constant  Value=0  OutDataTypeStr=fixdt(0,5,0)  SampleTime=-1
  Constant6 : Constant  Value=0  OutDataTypeStr=fixdt(0,4,0)  SampleTime=-1
  Constant7 : Constant  Value=0  OutDataTypeStr=fixdt(0,3,0)  SampleTime=-1
  Constant9 : Constant  Value=0  OutDataTypeStr=fixdt(0,2,0)  SampleTime=-1
  Data Type Conversion : DataTypeConversion  OutDataTypeStr=uint8  SaturateOnIntegerOverflow=off  RndMeth=Floor
  Data Type Conversion1 : DataTypeConversion  OutDataTypeStr=uint16  SaturateOnIntegerOverflow=off  RndMeth=Floor
  Data Type Conversion2 : DataTypeConversion  OutDataTypeStr=fixdt(0,6,0)  SaturateOnIntegerOverflow=off  RndMeth=Floor
  Data Type Conversion{3..5,8} (4 alike) : DataTypeConversion  OutDataTypeStr=fixdt(0,5,0)  SaturateOnIntegerOverflow=off  RndMeth=Floor
  Data Type Conversion6 : DataTypeConversion  OutDataTypeStr=fixdt(0,4,0)  SaturateOnIntegerOverflow=off  RndMeth=Floor
  Data Type Conversion7 : DataTypeConversion  OutDataTypeStr=fixdt(0,3,0)  SaturateOnIntegerOverflow=off  RndMeth=Floor
  Data Type Conversion9 : DataTypeConversion  OutDataTypeStr=fixdt(0,2,0)  SaturateOnIntegerOverflow=off  RndMeth=Floor
  Vector Concatenate{,1,3..7,9..10} (9 alike) : Concatenate
  Vector Concatenate11 : Concatenate  NumInputs=3
  Vector Concatenate2 : Concatenate  NumInputs=4
  Vector Concatenate8 : Concatenate  NumInputs=4
  Word to Bits : hdlsllib/Logic and Bit Operations/Word to Bits  maxWordLength=8
  Word to Bits1 : hdlsllib/Logic and Bit Operations/Word to Bits  maxWordLength=16
  Word to Bits2 : hdlsllib/Logic and Bit Operations/Word to Bits  maxWordLength=6
  Word to Bits{3..5,8} (4 alike) : hdlsllib/Logic and Bit Operations/Word to Bits  maxWordLength=5
  Word to Bits6 : hdlsllib/Logic and Bit Operations/Word to Bits  maxWordLength=4
  Word to Bits7 : hdlsllib/Logic and Bit Operations/Word to Bits  maxWordLength=3
  Word to Bits9 : hdlsllib/Logic and Bit Operations/Word to Bits  maxWordLength=2
  reg0 : Outport  SampleTime=8e-08
  reg1 : Outport  Port=2  SampleTime=8e-08
  reg2 : Outport  Port=3  SampleTime=8e-08
  reg3 : Outport  Port=4  SampleTime=8e-08
  wires:
  Word to Bits9/1 -> Vector Concatenate11/3
  Word to Bits8/1 -> Vector Concatenate10/2
  Word to Bits7/1 -> Vector Concatenate9/2
  Word to Bits6/1 -> Vector Concatenate7/2
  Word to Bits5/1 -> Vector Concatenate6/2
  Word to Bits4/1 -> Vector Concatenate5/2
  Word to Bits3/1 -> Vector Concatenate4/2
  Word to Bits2/1 -> Vector Concatenate3/2
  Word to Bits1/1 -> Vector Concatenate1/2
  Word to Bits/1 -> Vector Concatenate/2
  Vector Concatenate9/1 -> Vector Concatenate8/2
  Vector Concatenate8/1 -> Bits to Word3/1
  Vector Concatenate7/1 -> Vector Concatenate8/1
  Vector Concatenate6/1 -> Vector Concatenate2/4
  Vector Concatenate5/1 -> Vector Concatenate2/3
  Vector Concatenate4/1 -> Vector Concatenate2/2
  Vector Concatenate3/1 -> Vector Concatenate2/1
  Vector Concatenate2/1 -> Bits to Word2/1
  Vector Concatenate11/1 -> Vector Concatenate8/4
  Vector Concatenate10/1 -> Vector Concatenate8/3
  Vector Concatenate1/1 -> Bits to Word1/1
  Vector Concatenate/1 -> Bits to Word/1
  Data Type Conversion9/1 -> Word to Bits9/1
  Data Type Conversion8/1 -> Word to Bits8/1
  Data Type Conversion7/1 -> Word to Bits7/1
  Data Type Conversion6/1 -> Word to Bits6/1
  Data Type Conversion5/1 -> Word to Bits5/1
  Data Type Conversion4/1 -> Word to Bits4/1
  Data Type Conversion3/1 -> Word to Bits3/1
  Data Type Conversion2/1 -> Word to Bits2/1
  Data Type Conversion1/1 -> Word to Bits1/1
  Data Type Conversion/1 -> Word to Bits/1
  Constant9/1 -> Data Type Conversion9/1
  Constant8/1 -> Data Type Conversion8/1
  Constant7/1 -> Data Type Conversion7/1
  Constant6/1 -> Data Type Conversion6/1
  Constant5/1 -> Data Type Conversion5/1
  Constant4/1 -> Data Type Conversion4/1
  Constant3/1 -> Data Type Conversion3/1
  Constant2/1 -> Data Type Conversion2/1
  Constant1/1 -> Data Type Conversion1/1
  Constant/1 -> Data Type Conversion/1
  Bits to Word3/1 -> reg3/1
  Bits to Word2/1 -> reg2/1
  Bits to Word1/1 -> reg1/1
  Bits to Word/1 -> reg0/1
  mimo_number/1 -> Vector Concatenate11/2
  mimo_spacing/1 -> Vector Concatenate11/1
  cp_id/1 -> Vector Concatenate10/1
  bat_id/1 -> Vector Concatenate9/1
  scrambler_init/1 -> Vector Concatenate7/1
  concat_factor/1 -> Vector Concatenate6/1
  rep_number/1 -> Vector Concatenate5/1
  fec_rate/1 -> Vector Concatenate4/1
  block_size/1 -> Vector Concatenate3/1
  msg_duration/1 -> Vector Concatenate1/1
  psdu_size/1 -> Vector Concatenate/1

== system gm_HDLRx_vs/full_rx/h_rx_full/h_crc_rx ==
  data_in : Inport  OutDataTypeStr=boolean  SampleTime=1e-08
  ctrl_in : Inport  Port=2  SampleTime=1e-08
  General CRC Syndrome Detector HDL Optimized : commhdlcrc/General CRC Syndrome Detector HDL Optimized  Polynomial=headerCRCPoly  InitialState=1  DirectMethod=on  ReflectInput=off  ReflectCRCChecksum=off  FinalXORValue=0  SimulateUsing=Code generation
  Sample Control Bus Creator : whdlutilities/Sample Control Bus Creator
  Sample Control Bus Selector : whdlutilities/Sample Control Bus Selector  OutputSignals=start,end,valid
  Switch : Switch  Criteria=u2 ~= 0  OutDataTypeStr=boolean  SaturateOnIntegerOverflow=off  InputSameDT=off
  Unit Delay : UnitDelay  SampleTime=-1  HasFrameUpgradeWarning=on
  data_out : Outport  SampleTime=1e-08
  ctrl_out : Outport  Port=2  SampleTime=1e-08
  err : Outport  Port=3  SampleTime=1e-08
  wires:
  Unit Delay/1 -> Switch/3
  Switch/1 -> err/1, Unit Delay/1
  Sample Control Bus Selector/3 -> General CRC Syndrome Detector HDL Optimized/4  "<valid>"
  Sample Control Bus Selector/2 -> General CRC Syndrome Detector HDL Optimized/3  "<end>"
  Sample Control Bus Selector/1 -> General CRC Syndrome Detector HDL Optimized/2  "<start>"
  Sample Control Bus Creator/1 -> ctrl_out/1
  General CRC Syndrome Detector HDL Optimized/5 -> Switch/1
  General CRC Syndrome Detector HDL Optimized/4 -> Sample Control Bus Creator/3
  General CRC Syndrome Detector HDL Optimized/3 -> Sample Control Bus Creator/2, Switch/2
  General CRC Syndrome Detector HDL Optimized/2 -> Sample Control Bus Creator/1
  General CRC Syndrome Detector HDL Optimized/1 -> data_out/1
  ctrl_in/1 -> Sample Control Bus Selector/1
  data_in/1 -> General CRC Syndrome Detector HDL Optimized/1

== system gm_HDLRx_vs/full_rx/h_rx_full/h_remove_repetition ==
  data_in : Inport  OutDataTypeStr=int8  SampleTime=1e-08
  start_in : Inport  Port=2  OutDataTypeStr=boolean  SampleTime=1e-08
  HDL Counter : hdlsllib/Sources/HDL Counter  CountType=Count limited  CountInit=0  CountStep=1  CountMax=headerBitsPerFec-1  CountFromType=Initial value  CountFrom=0  CountResetPort=on  CountLoadPort=off  CountEnbPort=on  CountDirPort=off  CountHitOutputPort=on  CountDataType=Unsigned  CountWordLen=nextpow2(headerBitsPerFec)  CountFracLen=0  CountSampTime=1
  HDL Counter_term0 : Terminator
  Logical Operator : Logic  Operator=OR  AllPortsSameDT=off  OutDataTypeStr=boolean
  Sample Control Bus Creator : whdlutilities/Sample Control Bus Creator
  Switch : Switch  Criteria=u2 ~= 0  OutDataTypeStr=boolean  SaturateOnIntegerOverflow=off  InputSameDT=off
  Unit Delay{,1..7} (8 alike) : UnitDelay  SampleTime=-1  HasFrameUpgradeWarning=on
  data_out : Outport  SampleTime=1e-08
  ctrl_out : Outport  Port=2  SampleTime=1e-08
  wires:
  Unit Delay7/1 -> Sample Control Bus Creator/3
  Unit Delay6/1 -> Sample Control Bus Creator/1
  Unit Delay5/1 -> data_out/1
  Unit Delay4/1 -> Unit Delay5/1
  Unit Delay3/1 -> HDL Counter/1, Unit Delay6/1
  Unit Delay2/1 -> Switch/1
  Unit Delay1/1 -> Switch/2
  Unit Delay/1 -> Switch/3
  Switch/1 -> HDL Counter/2, Unit Delay/1, Unit Delay7/1
  Sample Control Bus Creator/1 -> ctrl_out/1
  Logical Operator/1 -> Unit Delay1/1
  HDL Counter/2 -> Sample Control Bus Creator/2, Logical Operator/2
  HDL Counter/1 -> HDL Counter_term0/1
  start_in/1 -> Unit Delay2/1, Unit Delay3/1, Logical Operator/1
  data_in/1 -> Unit Delay4/1
